simulink model "GNCModel"  (Simulink 7.9)
settings: Solver=FixedStepDiscrete  StartTime=0.0  StopTime=10.0  RelTol=1e-3
undefined symbols (not defined in the file): gcbh, rmidispblock
libraries: simulink x2, mptlib x1, rtweclib x1, dspadpt3 x1, mpclib x1, idelinklib_tgtpref x1
settings Model: Creator=spacekitteh  LastModifiedBy=spacekitteh
settings SolverCC: PositivePriorityOrder=on
settings DataIOCC: SaveOutput=off  SaveTime=off
settings OptimizationCC: InlineParams=on  InlineInvariantSignals=on  StateBitsets=on  DataBitsets=on  UseTempVars=on  ZeroExternalMemoryAtStartup=off  ZeroInternalMemoryAtStartup=off  NoFixptDivByZeroProtection=on  EfficientFloat2IntCast=on  OptimizeModelRefInitCode=on  LifeSpan=1
settings HardwareCC: ProdLargestAtomicInteger=Long  ProdLargestAtomicFloat=Double  ProdIntDivRoundTo=Zero  ProdEndianess=LittleEndian  ProdHWDeviceType=ARMCortex
settings RTWCC: SystemTargetFile=ert.tlc  TemplateMakefile=ert_default_tmf  Description=Embedded Coder  GenerateReport=on  RTWVerbose=off  ProcessScript=ert_make_rtw_hook  IncludeHyperlinkInReport=on  LaunchReport=on  GenerateTraceInfo=on  GenerateTraceReport=on  GenerateTraceReportSl=on  GenerateTraceReportSf=on  GenerateTraceReportEml=on
settings CodeAppCC: ForceParamTrailComments=on  IgnoreCustomStorageClasses=off  SimulinkDataObjDesc=on  CustomSymbolStrGlobalVar=rt$N$M  CustomSymbolStrType=$N$M  CustomSymbolStrFcn=$N$M$F  CustomSymbolStrMacro=$N$M  InsertBlockDesc=on
settings ERTTargetCC: CodeReplacementLibrary=ANSI_C  MultiwordLength=2048  GenerateSampleERTMain=on  IncludeMdlTerminateFcn=off  CombineSignalStateStructs=on  InlinedParameterPlacement=NonHierarchical  ERTCustomFileTemplate=example_file_process.tlc  ConvertIfToSwitch=off  SuppressUnreachableDefaultCases=off

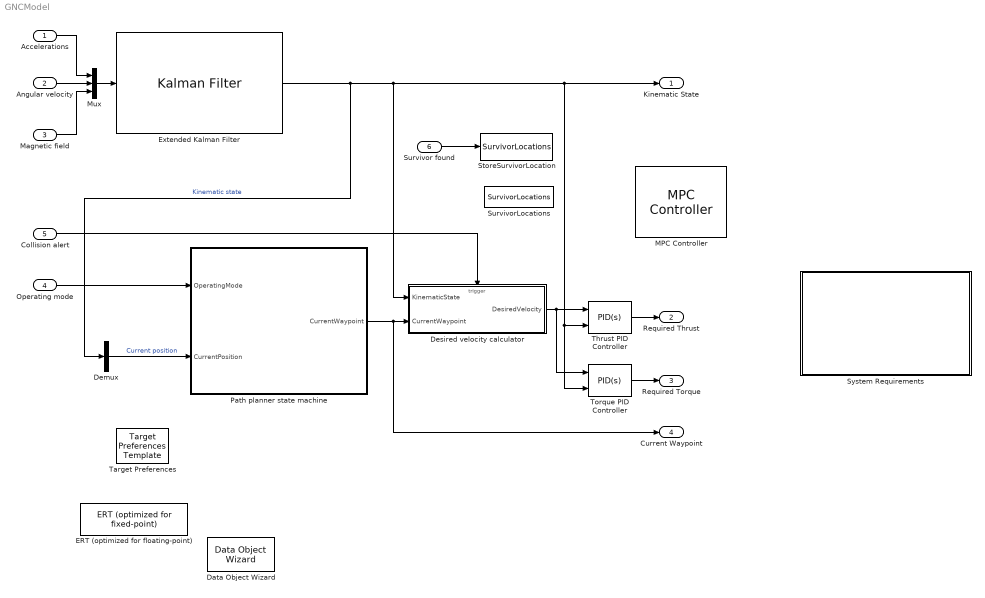
== system GNCModel ==
  Accelerations : Inport
  Angular velocity : Inport  Port=2
  Magnetic field : Inport  Port=3
  Operating mode : Inport  Port=4
  Collision alert : Inport  Port=5
  Survivor found : Inport  Port=6
  Data Object Wizard : mptlib/Data Object Wizard  Description=DOW
  Demux : Demux  Outputs=1
  Desired velocity calculator : Subsystem  TreatAsAtomicUnit=on
      settings: RTWFcnNameOpts=Use subsystem name  RTWFileNameOpts=Use function name
  ERT (optimized for floating-point) : rtweclib/Configuration Wizards/ERT (optimized for fixed-point)  ConfigMode=ERT (optimized for floating-point)  ConfigScript=rtwsampleconfig  InvokeBuild=off  ShowInLibBrowser=off
  Extended Kalman Filter : dspadpt3/Kalman Filter  num_targets=10  sourceEnable=Always  isReset=on  X=zeros([6, 1])  P=10*eye(6)  A=[1 0 1 0 0 0;0 1 0 1 0 0; 0 0 1 0 0 0; 0 0 0 1 0 0; 0 0 0 0 1 0; 0 0 0 0 0 1]  sourceMeasure=Specify via Dialog  H=[1 0 0 0 0 0; 0 1 0 0 0 0; 0 0 0 0 1 0; 0 0 0 0 0 1]  Q=0.05*eye(6)  R=eye(4)  isOutputEstMeasure=off  isOutputEstState=on  isOutputEstError=off  isOutputPrdMeasure=off  isOutputPrdState=off  isOutputPrdError=off
  MPC Controller : mpclib/MPC Controller  x0=[]  md_inport=on  mv_inport=off  lims_inport=off  switch_inport=off  ywt_inport=off  duwt_inport=off  rhoeps_inport=off  cost_outport=off  return_sequence=off  return_qpstatus=off  is_multiple=0  enable_value=0  n_mv=0  n_mo=0  n_md=0  n_ts=0  is_designfromscratch=0  ref_from_ws=off  ref_signal_name=[]  ref_preview=on  md_from_ws=off  md_signal_name=[]  md_preview=on  from_project=off  project_file=MPCtask.mat
  Mux : Mux  Inputs=3
  Path planner state machine : Stateflow chart  TreatAsAtomicUnit=on
  StoreSurvivorLocation : DataStoreWrite  DataStoreName=SurvivorLocations
  SurvivorLocations : DataStoreMemory  DataStoreName=SurvivorLocations  ReadBeforeWriteMsg=warning  WriteAfterWriteMsg=warning  WriteAfterReadMsg=warning
  System Requirements : Subsystem  LoadFcn=rmidispblock('load',gcbh)  mask(System Requirements){id=SystemReq, title=System Requirements}
      mask prompts: title "Block Title"
      mask help: Lists the requirements for the current model.
      mask init:
      | id = 'SystemReq';
      | [w,h] = rmidispblock('display',gcbh);
      settings: CopyFcn=rmidispblock('create',gcbh)  DeleteFcn=rmidispblock('delete',gcbh)  ModelCloseFcn=rmidispblock('close',gcbh)  PreSaveFcn=rmidispblock('close',gcbh)  PostSaveFcn=rmidispblock('open',gcbh)  OpenFcn=rmidispblock('open',gcbh)  MoveFcn=rmidispblock('move',gcbh)
      mask Help: helpview(fullfile(docroot,'toolbox','slvnv','slvnv.map'),'systemrequirements')
      mask Display:
      | text(w/2,h-4,rmidispblock('title',gcbh),'horizontalAlignment','center','verticalAlignment','top')
      | text(w/2,h/2,'<No Requirements in System>','horizontalAlignment','center','verticalAlignment','top')
  Target Preferences : idelinklib_tgtpref/Target Preferences Template  Tag=eclipseidetgtpref  library=off
  Thrust PID Controller : simulink/Continuous/PID Controller (2DOF)  Controller=PID  TimeDomain=Continuous-time  SampleTime=1  IntegratorMethod=Forward Euler  FilterMethod=Forward Euler  Form=Parallel  P=1  I=1  D=0  N=100  b=1  c=1  InitialConditionSource=internal  InitialConditionForIntegrator=0  InitialConditionForFilter=0  ExternalReset=none  LimitOutput=off  UpperSaturationLimit=inf  LowerSaturationLimit=-inf  LinearizeAsGain=off  AntiWindupMode=none  Kb=1  TrackingMode=off  Kt=1  PParamMin=[]  PParamMax=[]  IParamMin=[]  IParamMax=[]  DParamMin=[]  DParamMax=[]  NParamMin=[]  NParamMax=[]  bParamMin=[]  bParamMax=[]  cParamMin=[]  cParamMax=[]  KbParamMin=[]  KbParamMax=[]  KtParamMin=[]  KtParamMax=[]  POutMin=[]  POutMax=[]  IOutMin=[]  IOutMax=[]  DOutMin=[]  DOutMax=[]  NOutMin=[]  NOutMax=[]  bOutMin=[]  bOutMax=[]  cOutMin=[]  cOutMax=[]  KbOutMin=[]  KbOutMax=[]  KtOutMin=[]  KtOutMax=[]  IntegratorOutMin=[]  IntegratorOutMax=[]  FilterOutMin=[]  FilterOutMax=[]  SumOutMin=[]  SumOutMax=[]  Sum1OutMin=[]  Sum1OutMax=[]  Sum2OutMin=[]  Sum2OutMax=[]  Sum3OutMin=[]  Sum3OutMax=[]  SumI1OutMin=[]  SumI1OutMax=[]  SumI2OutMin=[]  SumI2OutMax=[]  SumI3OutMin=[]  SumI3OutMax=[]  SumDOutMin=[]  SumDOutMax=[]  SaturationOutMin=[]  SaturationOutMax=[]  IntegratorContinuousStateAttributes=''  IntegratorStateMustResolveToSignalObject=off  IntegratorRTWStateStorageClass=Auto  FilterContinuousStateAttributes=''  FilterStateMustResolveToSignalObject=off  FilterRTWStateStorageClass=Auto
  Torque PID Controller : simulink/Continuous/PID Controller (2DOF)  Controller=PID  TimeDomain=Continuous-time  SampleTime=1  IntegratorMethod=Forward Euler  FilterMethod=Forward Euler  Form=Parallel  P=1  I=1  D=0  N=100  b=1  c=1  InitialConditionSource=internal  InitialConditionForIntegrator=0  InitialConditionForFilter=0  ExternalReset=none  LimitOutput=off  UpperSaturationLimit=inf  LowerSaturationLimit=-inf  LinearizeAsGain=off  AntiWindupMode=none  Kb=1  TrackingMode=off  Kt=1  PParamMin=[]  PParamMax=[]  IParamMin=[]  IParamMax=[]  DParamMin=[]  DParamMax=[]  NParamMin=[]  NParamMax=[]  bParamMin=[]  bParamMax=[]  cParamMin=[]  cParamMax=[]  KbParamMin=[]  KbParamMax=[]  KtParamMin=[]  KtParamMax=[]  POutMin=[]  POutMax=[]  IOutMin=[]  IOutMax=[]  DOutMin=[]  DOutMax=[]  NOutMin=[]  NOutMax=[]  bOutMin=[]  bOutMax=[]  cOutMin=[]  cOutMax=[]  KbOutMin=[]  KbOutMax=[]  KtOutMin=[]  KtOutMax=[]  IntegratorOutMin=[]  IntegratorOutMax=[]  FilterOutMin=[]  FilterOutMax=[]  SumOutMin=[]  SumOutMax=[]  Sum1OutMin=[]  Sum1OutMax=[]  Sum2OutMin=[]  Sum2OutMax=[]  Sum3OutMin=[]  Sum3OutMax=[]  SumI1OutMin=[]  SumI1OutMax=[]  SumI2OutMin=[]  SumI2OutMax=[]  SumI3OutMin=[]  SumI3OutMax=[]  SumDOutMin=[]  SumDOutMax=[]  SaturationOutMin=[]  SaturationOutMax=[]  IntegratorContinuousStateAttributes=''  IntegratorStateMustResolveToSignalObject=off  IntegratorRTWStateStorageClass=Auto  FilterContinuousStateAttributes=''  FilterStateMustResolveToSignalObject=off  FilterRTWStateStorageClass=Auto
  Kinematic State : Outport
  Required Thrust : Outport  Port=2
  Required Torque : Outport  Port=3
  Current Waypoint : Outport  Port=4
  wires:
  Accelerations/1 -> Mux/1
  Angular velocity/1 -> Mux/2
  Magnetic field/1 -> Mux/3
  Mux/1 -> Extended Kalman Filter/1
  Extended Kalman Filter/1 -> Demux/1, Desired velocity calculator/1(KinematicState), Kinematic State/1, Thrust PID Controller/2, Torque PID Controller/2  "Kinematic state"
  Demux/1 -> Path planner state machine/2(CurrentPosition)  "Current position"
  Operating mode/1 -> Path planner state machine/1(OperatingMode)
  Path planner state machine/1(CurrentWaypoint) -> Desired velocity calculator/2(CurrentWaypoint), Current Waypoint/1
  Desired velocity calculator/1(DesiredVelocity) -> Thrust PID Controller/1, Torque PID Controller/1
  Thrust PID Controller/1 -> Required Thrust/1
  Torque PID Controller/1 -> Required Torque/1
  Collision alert/1 -> Desired velocity calculator/Trigger
  Survivor found/1 -> StoreSurvivorLocation/1

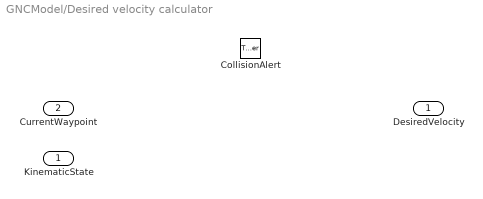
== system GNCModel/Desired velocity calculator ==
  KinematicState : Inport
  CurrentWaypoint : Inport  Port=2
  CollisionAlert : TriggerPort  PortDimensions=1
  DesiredVelocity : Outport

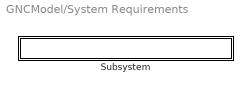
== system GNCModel/System Requirements ==
  Subsystem : Subsystem  mask{label=0, index=1}
      mask init:
      | label = rmidispblock('label',index);
      settings: OpenFcn=rmidispblock('openReq',gcbh);
      mask Display: text(0,0,label,'horizontalAlignment','left','verticalAlignment','bottom')

== system GNCModel/System Requirements/Subsystem ==

== stateflow chart Path planner state machine ==
  state SearchingForSurvivor
  (default) -> (junction 4)
  data: OperatingMode input int8; CurrentPosition input double; CurrentWaypoint output double(3)
